simulink model "MPC_f2s_sim"  (R2022b)
settings: Solver=FixedStepAuto  StartTime=0.0  StopTime=50  FixedStep=0.01  RelTol=1e-3
model workspace (MAT data in the model file):
  L = 2.9
values from neighbouring files (symbols this model uses):
  map_ori = ~map    [DWA.m]    (also in preprocessing.m = sysu; rrt_star.m = im2bw(imread('map_ori.png')))
  out_ = zeros(600,1200,3)    [generate_out_for_simulink.m]    (also in preprocessing.m)
  traj_gaobo = traj_gaobo'    [DWA.m]
undefined symbols (not defined in the file or in its folder): gray
settings Model: Creator=13349  LastModifiedBy=ps
settings SolverCC: AlgebraicLoopSolver=TrustRegion
settings DebuggingCC: UnconnectedInputMsg=warning  UnconnectedOutputMsg=warning  UnconnectedLineMsg=warning  ArithmeticOperatorsInVariantConditions=warning
settings ModelReferenceCC: EnableRefExpFcnMdlSchedulingChecks=on
settings SFSimCC: CustomCodeUndefinedFunction=UseInterfaceOnly

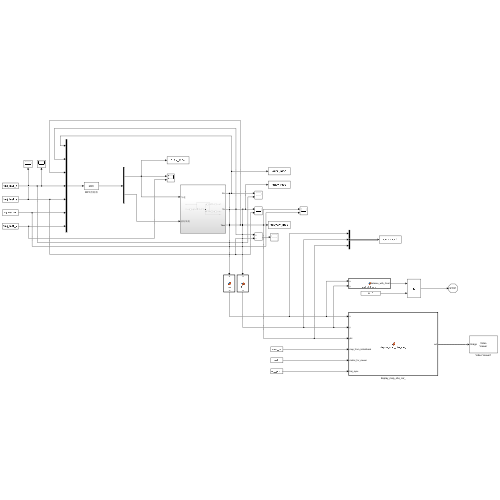
[thumbnail: Simulink's stored preview of the top-level diagram]
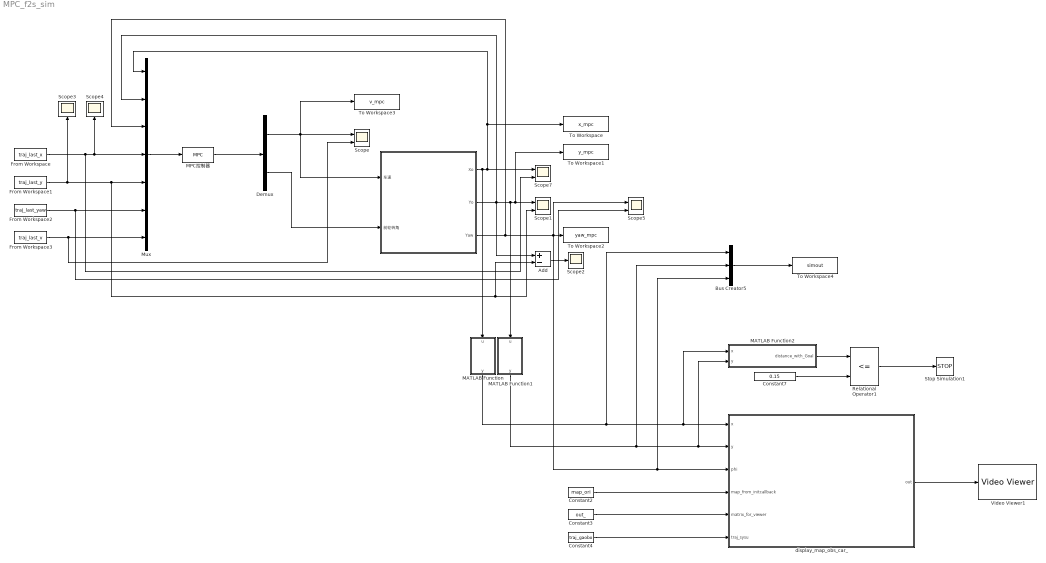
== system MPC_f2s_sim ==
  " " : Subsystem
  Add : Sum  Inputs=+-
  Bus Creator5 : BusCreator  Inputs=3
  Constant2 : Constant  Value=map_ori
  Constant3 : Constant  Value=out_
  Constant4 : Constant  Value=traj_gaobo
  Constant7 : Constant  Value=0.15
  Demux : Demux  Outputs=2
  From Workspace : FromWorkspace  VariableName=traj_last_x
  From Workspace1 : FromWorkspace  VariableName=traj_last_y
  From Workspace2 : FromWorkspace  VariableName=traj_last_yaw
  From Workspace3 : FromWorkspace  VariableName=traj_last_v
  MATLAB Function : MATLAB Function  TreatAsAtomicUnit=on
  MATLAB Function1 : MATLAB Function  TreatAsAtomicUnit=on
  MATLAB Function2 : MATLAB Function  TreatAsAtomicUnit=on
  MPC控制器 : S-Function  InitFcn=[80,520,0]  FunctionName=MPC  SFunctionDeploymentMode=off  EnableBusSupport=off
  Mux : Mux  InitFcn=u = [1.095330803283442e+02; 10.303616806213880; 0.0207795418315176; 1.095330803283442e+02; 10.303616806213880; 0.0207795418315176; 13.0];  Inputs=7
  Relational Operator1 : RelationalOperator  Operator=<=  OutDataTypeStr=boolean  InputSameDT=off
  Scope{,1,5,7} (4 alike) : Scope  NumInputPorts=2
  Scope2 : Scope
  Scope3 : Scope
  Scope4 : Scope
  Stop Simulation1 : Stop
  To Workspace : ToWorkspace  VariableName=x_mpc  SaveFormat=Timeseries  SampleTime=-1
  To Workspace1 : ToWorkspace  VariableName=y_mpc  SaveFormat=Timeseries  SampleTime=-1
  To Workspace2 : ToWorkspace  VariableName=yaw_mpc  SaveFormat=Timeseries  SampleTime=-1
  To Workspace3 : ToWorkspace  VariableName=v_mpc  SaveFormat=Timeseries  SampleTime=-1
  To Workspace4 : ToWorkspace  VariableName=simout  SaveFormat=Timeseries  SampleTime=-1
  Video Viewer1 : VideoViewer  colormapValue=gray(256)  FigPos=[675 1143.33333333333 1539.33333333333 646.666666666667]
  display_map_obs_car_ : MATLAB Function  TreatAsAtomicUnit=on
  wires:
  " "/1(Xo) -> Scope7/1, Mux/1, To Workspace/1, MATLAB Function/1(u)
  " "/2(Yo) -> Scope1/1, To Workspace1/1, MATLAB Function1/1(u), Mux/2, Add/1
  " "/3(Yaw) -> Mux/3, Bus Creator5/3, display_map_obs_car_/3(phi), Scope5/1, To Workspace2/1
  Mux/1 -> MPC控制器/1
  MPC控制器/1 -> Demux/1
  Demux/2 -> " "/2(前轮转角)
  Demux/1 -> " "/1(车速), To Workspace3/1, Scope/1
  Add/1 -> Scope2/1
  From Workspace/1 -> Scope7/2, Scope4/1, Mux/4
  From Workspace3/1 -> Scope/2, Mux/7
  From Workspace2/1 -> Scope5/2, Mux/6
  From Workspace1/1 -> Scope3/1, Add/2, Scope1/2, Mux/5
  MATLAB Function/1(y) -> MATLAB Function2/1(x), display_map_obs_car_/1(x), Bus Creator5/1
  MATLAB Function1/1(y) -> MATLAB Function2/2(y), display_map_obs_car_/2(y), Bus Creator5/2
  Constant4/1 -> display_map_obs_car_/6(traj_sysu)
  Constant2/1 -> display_map_obs_car_/4(map_from_initcallback)
  Constant3/1 -> display_map_obs_car_/5(matrix_for_viewer)
  display_map_obs_car_/1(out) -> Video Viewer1/1
  MATLAB Function2/1(distance_with_Goal) -> Relational Operator1/1
  Constant7/1 -> Relational Operator1/2
  Bus Creator5/1 -> To Workspace4/1
  Relational Operator1/1 -> Stop Simulation1/1

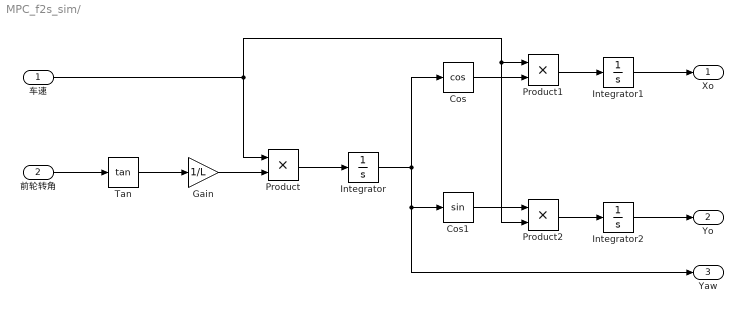
== system MPC_f2s_sim/  ==
  车速 : Inport
  前轮转角 : Inport  Port=2
  Cos : Trigonometry  Operator=cos
  Cos1 : Trigonometry
  Gain : Gain  Gain=1/L
  Integrator : Integrator
  Integrator1 : Integrator
  Integrator2 : Integrator
  Product : Product
  Product1 : Product
  Product2 : Product
  Tan : Trigonometry  Operator=tan
  Xo : Outport
  Yo : Outport  Port=2
  Yaw : Outport  Port=3
  wires:
  Integrator/1 -> Yaw/1, Cos1/1, Cos/1
  Gain/1 -> Product/2
  前轮转角/1 -> Tan/1
  Cos/1 -> Product1/2
  Integrator1/1 -> Xo/1
  Tan/1 -> Gain/1
  Cos1/1 -> Product2/1
  车速/1 -> Product2/2, Product1/1, Product/1
  Integrator2/1 -> Yo/1
  Product/1 -> Integrator/1
  Product1/1 -> Integrator1/1
  Product2/1 -> Integrator2/1

== matlab function MPC_f2s_sim/MATLAB Function1 ==
  data: u input; y output
function y = fcn(u)

y = u * 0.01 + 0.8;

end

== matlab function MPC_f2s_sim/display_map_obs_car_ ==
  settings: updateMethod=DISCRETE
  data: x input; y input; phi input; out output size=600,1200,3; map_from_initcallback input size=600,1200; matrix_for_viewer input; traj_sysu input
function out = display_map_obs_car_(x,y,phi,map_from_initcallback,matrix_for_viewer,traj_sysu)
    persistent data;
    persistent times;
    if isempty(data)
        times=1;
    else
        times=times+1;
    end
    traj_sysu(1,:) = traj_sysu(1,:)*0.01;
    traj_sysu(2,:) = traj_sysu(2,:)*0.01;
    % 地图长12m 宽6m   车长0.12 车宽0.06
    resolution = 0.01;
    map_long=12;
    map_wide=6;

    car_long=0.12;
    car_wide=0.06;

%     % 可视化地图
%     figure;
%     imagesc(map);%imagesc 可以将矩阵或数组的值映射到颜色图像中
%     colormap(flipud(gray));%colormap 将数据值映射到颜色空间中 colormap(flipud(gray)) 来设置颜色映射表为灰度图像。
    map=map_from_initcallback;    
    out=matrix_for_viewer;
    number_path=size(traj_sysu,2);
    for tmp=1:number_path
        traj_sysu_index=real2map([traj_sysu(1,tmp),traj_sysu(2,tmp)],map_wide,resolution);
        out(fix(traj_sysu_index(1)+1/2),fix(traj_sysu_index(2)+1/2),:)=[0,0,0];
    end
    x_now=x;%m  real视野坐标系,横着往右
    y_now=y;%m  real视野坐标系,竖着往上
    map_coord=real2map([x_now,y_now],map_wide,resolution);
    if isempty(data)
        data = zeros(99999, 2);
    else
        data(round(times/10)+1,:) = [map_coord(1),map_coord(2)];
        for times_disp_tmp=1:round(times/10)
            tmp_Data=data(times_disp_tmp,:);
            tmp_Data_next=data(times_disp_tmp+1,:);
%             out(round(tmp_Data(1,1)+1/2),round(tmp_Data(1,2)+1/2),:)=[0,0,1];

    
            vector=tmp_Data_next-tmp_Data;
            for t=0:0.025:1
                    new_point=tmp_Data+t*vector;
                    out(round(new_point(1)+1/2),round(new_point(2)+1/2),:)=[0,0,1];
                    out(round(new_point(1)+1/2),round(new_point(2)+1/2)-1,:)=[0,0,1];
                    out(round(new_point(1)+1/2),round(new_point(2)+1/2)+1,:)=[0,0,1];
            end

        end
    end



   
%     occ_or_not=get_occ_or_not(map_coord,map,resolution)
    occ_or_not=get_occ_or_not_Real([x_now,y_now],map_wide,map,resolution);
    l = car_long / resolution;
    w = car_wide / resolution;
    phi = phi; 




out=display_car(map_coord,phi,l,w,map,out);

%     axis equal;
%     axis off;
end

function occ_or_not=get_occ_or_not_Real(x_y,map_wide,map,resolution)
%round四舍五入 
map_coord=real2map(x_y,map_wide,resolution);
if(round(map_coord(1)+1/2)<1) ||(round(map_coord(1)+1/2)>600) ||(round(map_coord(2)+1/2)<1) ||(round(map_coord(2)+1/2)>1200)
    x_y
    disp('out of map');
end
 occ_or_not=map(round(map_coord(1)+1/2),round(map_coord(2)+1/2));
end
function occ_or_not=get_occ_or_not_map(map_coord,map,resolution)
%round四舍五入 
if(round(map_coord(1)+1/2)<1) ||(round(map_coord(1)+1/2)>600) ||(round(map_coord(2)+1/2)<1) ||(round(map_coord(2)+1/2)>1200)
    disp('out of map');
end
 occ_or_not=map(round(map_coord(1)+1/2),round(map_coord(2)+1/2));
end
function map_coord=real2map(x_y,map_wide,resolution)
    %地图向下是正x 向右是正y，
    % 因此在map上显示赛道小车障碍物的时候map_y直接取real世界的x, map_x需要把real_y反向并弄个静差
    map_coord=zeros(1,2);
    map_coord(1)=map_wide/ resolution-x_y(2)/ resolution;
    map_coord(2)=x_y(1)/ resolution ;
end

function matrix_for_viewer_new=display_car(map_coord,phi,l,w,map,matrix_for_viewer)
    %display是向右是x正，向下是y正
    pts = [
        map_coord(1)- [sin(phi)*l-cos(phi)*w, sin(phi)*l+cos(phi)*w,-sin(phi)*l+cos(phi)*w,-sin(phi)*l-cos(phi)*w]
        map_coord(2) + [cos(phi)*l+sin(phi)*w, cos(phi)*l-sin(phi)*w,-cos(phi)*l-sin(phi)*w,-cos(phi)*l+sin(phi)*w]
        
    ];
    map_index1=[round(pts(1,1)+1/2),round(pts(2,1)+1/2)];
    map_index2=[round(pts(1,2)+1/2),round(pts(2,2)+1/2)];
    map_index3=[round(pts(1,3)+1/2),round(pts(2,3)+1/2)];
    map_index4=[round(pts(1,4)+1/2),round(pts(2,4)+1/2)];

    matrix_for_viewer_new=matrix_for_viewer;
    %凸包，边缘线无碰撞则整体无碰撞
    have_somewhere_occ=0;
    vector_A_B=[map_index2(1)-map_index1(1),map_index2(2)-map_index1(2)];
    vector_A_D=[map_index4(1)-map_index1(1),map_index4(2)-map_index1(2)];
    for t1=0:0.025:1
        for t2=0:0.025:1
            new_point=map_index1+t1*vector_A_B+t2*vector_A_D;
            matrix_for_viewer_new(round(new_point(1)+0.5),round(new_point(2)+0.5),:)=[1,0,0];
            occ_or_not=map(round(new_point(1)+0.5),round(new_point(2)+0.5));
            if(occ_or_not==1)
               have_somewhere_occ=1;
           end
        end
    end
    if(have_somewhere_occ==1)
%         disp("collision!!");
    end
end

== matlab function MPC_f2s_sim/MATLAB Function ==
  data: u input; y output
function y = fcn(u)

y = u * 0.01 + 0.8;

end

== matlab function MPC_f2s_sim/MATLAB Function2 ==
  data: x input; distance_with_Goal output; y input
function distance_with_Goal = cal_distance(x,y)
distance_with_Goal=sqrt((x-11.3)*(x-11.3)+(y-4.5)*(y-4.5));
